simulink model "Utkarsh_2005574_W2_P3"  (R2020b)
settings: Solver=VariableStepAuto  StartTime=0.0  StopTime=120  RelTol=1e-3
PostLoadFcn:
  | M=1000;
  | b=50;
  | u=500;
  | 
  | Kp=19.9969;
  | Ki=0.34998;
  | Ts=3.36;
InitFcn:
  | M=1000;
  | b=50;
  | u=500;
  | 
  | Kp=19.9969;
  | Ki=0.34998;
  | Ts=3.36;
settings Model: Creator=home  LastModifiedBy=home
settings DebuggingCC: ModelReferenceExtraNoncontSigs=none

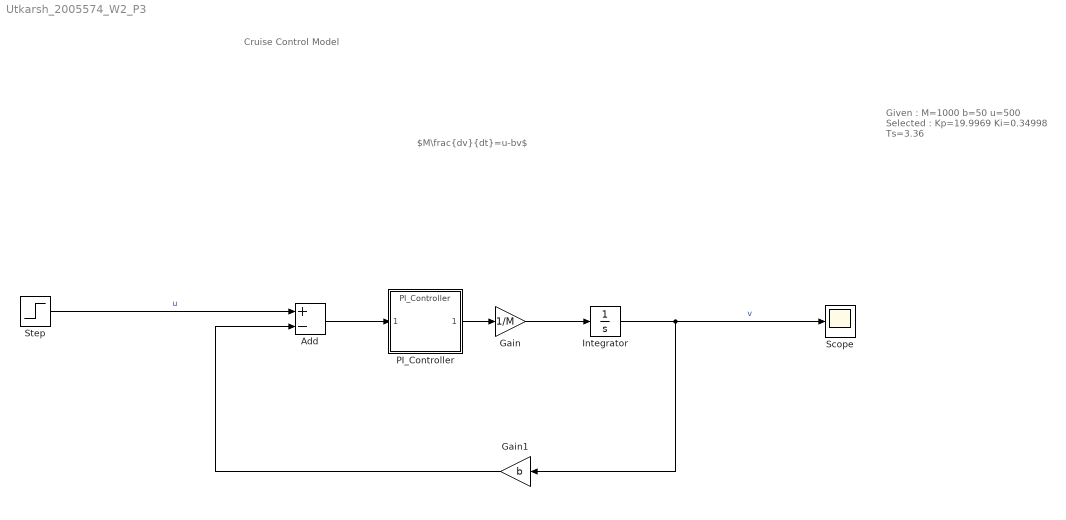
== system Utkarsh_2005574_W2_P3 ==
  note: Given :
      | M=1000
      | b=50
      | u=500
      |
      | Selected :
      | Kp=19.9969
      | Ki=0.34998
      | Ts=3.36
  note: $M\frac{dv}{dt}=u-bv$
  note: Cruise Control Model
  Add : Sum  Inputs=+-
  Gain : Gain  Gain=1/M
  Gain1 : Gain  Gain=b
  Integrator : Integrator
  PI_Controller : ModelReference  ModelNameDialog=PI_Controller  SimulationMode=Normal  ModelReferenceVersion=1.2
  Scope : Scope
  Step : Step  Time=0  After=u  SampleTime=0
  wires:
  Integrator/1 -> Scope/1, Gain1/1  "v"
  Step/1 -> Add/1  "u"
  Gain/1 -> Integrator/1
  Gain1/1 -> Add/2
  Add/1 -> PI_Controller/1
  PI_Controller/1 -> Gain/1
